simulink model "ISC_laboratorio_02_ex1"  (R2019a)
settings: Solver=FixedStepAuto  StartTime=0.0  StopTime=20  FixedStep=1e-2  RelTol=1e-3
settings Model: Creator=guilh  LastModifiedBy=guilh
settings DataIOCC: SaveOutput=off  SignalLogging=off  DSMLogging=off  ReturnWorkspaceOutputs=off  TimeSaveName=t

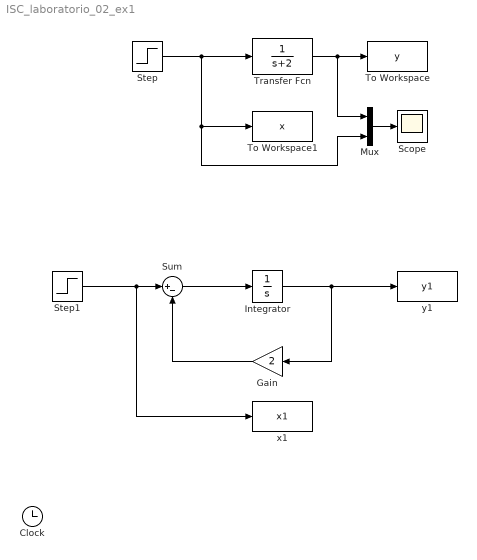
== system ISC_laboratorio_02_ex1 ==
  Clock : Clock
  Gain : Gain  Gain=2
  Integrator : Integrator  InitialCondition=1
  Mux : Mux  Inputs=2
  Scope : Scope
  Step : Step  Time=0  After=2  SampleTime=0
  Step1 : Step  Time=0  Before=2  After=0  SampleTime=0
  Sum : Sum  Inputs=|+-
  To Workspace : ToWorkspace  VariableName=y  SampleTime=-1
  To Workspace1 : ToWorkspace  VariableName=x  SampleTime=-1
  Transfer Fcn : TransferFcn  Denominator=[1 2]
  x1 : ToWorkspace  VariableName=x1  SampleTime=-1
  y1 : ToWorkspace  VariableName=y1  SampleTime=-1
  wires:
  Step/1 -> Mux/2, To Workspace1/1, Transfer Fcn/1
  Mux/1 -> Scope/1
  Transfer Fcn/1 -> Mux/1, To Workspace/1
  Integrator/1 -> Gain/1, y1/1
  Gain/1 -> Sum/2
  Sum/1 -> Integrator/1
  Step1/1 -> x1/1, Sum/1
